simulink model "pulse_heating_single_pack_v03"  (R2025b)
settings: Solver=ode23t  StartTime=0.0  StopTime=1  MaxStep=1e-4  RelTol=1e-3
undefined symbols (not defined in the file or in its folder): DiscIntNeverNeededParam
libraries: fl_lib x6, nesl_utility x5, ee_lib x4, batt_lib x1
settings Model: Creator=ADMIN  LastModifiedBy=ADMIN

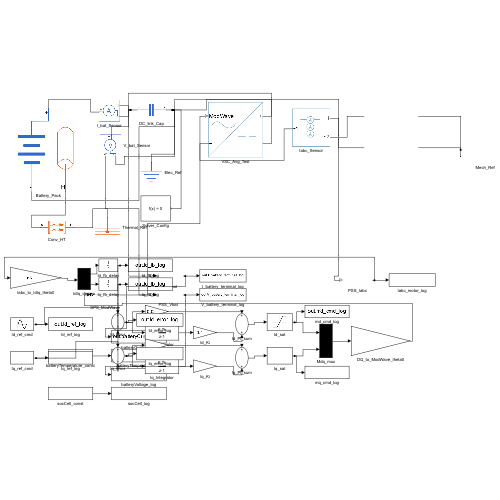
[thumbnail: Simulink's stored preview of the top-level diagram]
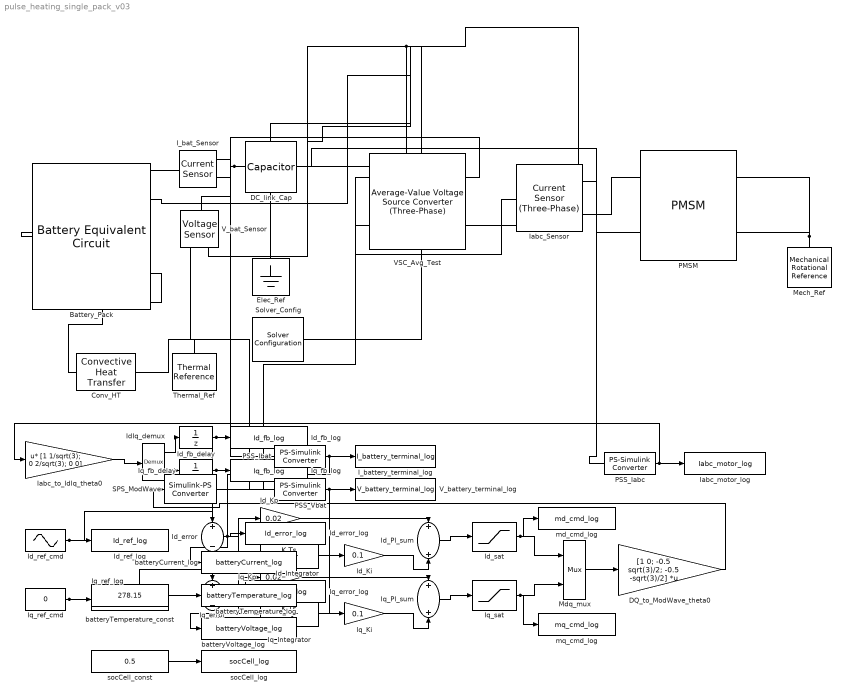
== system pulse_heating_single_pack_v03 ==
  Battery_Pack : batt_lib/Cells/Battery Equivalent Circuit  BatteryCapacity=27 A*hr  ThermalModel=simscape.battery.enum.cells.BatteryThermalModel.LumpedThermalMass  ExtrapolationMethod=simscape.enum.extrapolation.nearest  SOCBreakpoints=[0 0.1 0.25 0.5 0.75 0.9 1]  TemperatureBreakpoints=[278 293 313] K  OpenCircuitVoltage=[757.2312 770.256 784.8792 801.9432 847.9944 880.7832 905.6448] V  OpenCircuitVoltageThermal=[753.84 756 758.16;766.8 771.12 768.96;781.92 784.08 786.24;801.36 801.36 803.52;844.56 848.88 851.04;879.12 881.28 881.28;905.04 905.04 905.04] V  VoltageRange=[0, inf] V  HysteresisModel=simscape.battery.enum.cells.HysteresisModel.none  MaximumHysteresisVoltage=[0, 0, 0, 0, 0, 0, 0] V  InstantaneousHysteresisVoltage=[0, 0, 0, 0, 0, 0, 0] V  HysteresisRate=0.1  MaximumHysteresisVoltageThermal=[0, 0, 0; 0, 0, 0; 0, 0, 0; 0, 0, 0; 0, 0, 0; 0, 0, 0; 0, 0, 0] V  InstantaneousHysteresisVoltageThermal=[0, 0, 0; 0, 0, 0; 0, 0, 0; 0, 0, 0; 0, 0, 0; 0, 0, 0; 0, 0, 0] V  HysteresisRateThermal=0.1  ResistanceSOCBreakpoints=[0, .1, .25, .5, .75, .9, 1]  ResistanceTemperatureBreakpoints=[278, 293, 313] K  ResistanceCurrentBreakpoints=[-1 0 1] A  CurrentDependence=simscape.battery.enum.cells.CurrentDependence.Disabled  R0=[1.836 1.836 1.8792 1.7712 1.7928 1.836 1.836] Ohm  R0I=[2.5272 1.836 1.944;2.376 1.836 1.944;2.4624 1.8792 1.9872;2.3112 1.7712 1.9008;2.3112 1.7928 1.9656;2.4408 1.836 1.9224;2.5056 1.836 1.9224] Ohm  R0Thermal=[2.5272 1.836 1.944;2.376 1.836 1.944;2.4624 1.8792 1.9872;2.3112 1.7712 1.9008;2.3112 1.7928 1.9656;2.4408 1.836 1.9224;2.5056 1.836 1.9224] Ohm  R0ThermalI=repmat([2.5272 1.836 1.944;2.376 1.836 1.944;2.4624 1.8792 1.9872;2.3112 1.7712 1.9008;2.3112 1.7928 1.9656;2.4408 1.836 1.9224;2.5056 1.836 1.9224], 1, 1, 3) Ohm  DischargeR0=[.0085, .0085, .0087, .0082, .0083, .0085, .0085] Ohm  ChargeR0=[.0085, .0085, .0087, .0082, .0083, .0085, .0085] Ohm  ChargeR0Thermal=[.0117, .0085, .009; .011, .0085, .009; .0114, .0087, .0092; .0107, .0082, .0088; .0107, .0083, .0091; .0113, .0085, .0089; .0116, .0085, .0089] Ohm  DischargeR0Thermal=[.0117, .0085, .009; .011, .0085, .009; .0114, .0087, .0092; .0107, .0082, .0088; .0107, .0083, .0091; .0113, .0085, .0089; .0116, .0085, .0089] Ohm  RCPairs=simscape.battery.enum.cells.RCPairs.noDynamics  R1=[.0029, .0024, .0026, .0016, .0023, .0018, .0017] Ohm  Tau1=[36, 45, 105, 29, 77, 33, 39] s  R2=[.0029, .0024, .0026, .0016, .0023, .0018, .0017] Ohm  Tau2=[36, 45, 105, 29, 77, 33, 39] s  R3=[.0029, .0024, .0026, .0016, .0023, .0018, .0017] Ohm  Tau3=[36, 45, 105, 29, 77, 33, 39] s  R1I=[.0109, .0029, .0013; .0069, .0024, .0012; .0047, .0026, .0013; .0034, .0016, .001; .0033, .0023, .0014; .0033, .0018, .0011; .0028, .0017, .0011] Ohm  Tau1I=[20, 36, 39; 31, 45, 39; 109, 105, 61; 36, 29, 26; 59, 77, 67; 40, 33, 29; 25, 39, 33] s  R2I=[.0109, .0029, .0013; .0069, .0024, .0012; .0047, .0026, .0013; .0034, .0016, .001; .0033, .0023, .0014; .0033, .0018, .0011; .0028, .0017, .0011] Ohm  Tau2I=[20, 36, 39; 31, 45, 39; 109, 105, 61; 36, 29, 26; 59, 77, 67; 40, 33, 29; 25, 39, 33] s  R3I=[.0109, .0029, .0013; .0069, .0024, .0012; .0047, .0026, .0013; .0034, .0016, .001; .0033, .0023, .0014; .0033, .0018, .0011; .0028, .0017, .0011] Ohm  Tau3I=[20, 36, 39; 31, 45, 39; 109, 105, 61; 36, 29, 26; 59, 77, 67; 40, 33, 29; 25, 39, 33] s  DischargeR1=[0.6264 0.5184 0.5616 0.3456 0.4968 0.3888 0.3672] Ohm  DischargeTau1=[36 45 105 29 77 33 39] s  ChargeR1=[0.6264 0.5184 0.5616 0.3456 0.4968 0.3888 0.3672] Ohm  ChargeTau1=[36 45 105 29 77 33 39] s  DischargeR2=[0.6264 0.5184 0.5616 0.3456 0.4968 0.3888 0.3672] Ohm  DischargeTau2=[36 45 105 29 77 33 39] s  ChargeR2=[0.6264 0.5184 0.5616 0.3456 0.4968 0.3888 0.3672] Ohm  ChargeTau2=[36 45 105 29 77 33 39] s  DischargeR3=[0.6264 0.5184 0.5616 0.3456 0.4968 0.3888 0.3672] Ohm  DischargeTau3=[36 45 105 29 77 33 39] s  ChargeR3=[0.6264 0.5184 0.5616 0.3456 0.4968 0.3888 0.3672] Ohm  ChargeTau3=[36 45 105 29 77 33 39] s  R1Thermal=[.0109, .0029, .0013; .0069, .0024, .0012; .0047, .0026, .0013; .0034, .0016, .001; .0033, .0023, .0014; .0033, .0018, .0011; .0028, .0017, .0011] Ohm  Tau1Thermal=[20, 36, 39; 31, 45, 39; 109, 105, 61; 36, 29, 26; 59, 77, 67; 40, 33, 29; 25, 39, 33] s  R2Thermal=[.0109, .0029, .0013; .0069, .0024, .0012; .0047, .0026, .0013; .0034, .0016, .001; .0033, .0023, .0014; .0033, .0018, .0011; .0028, .0017, .0011] Ohm  Tau2Thermal=[20, 36, 39; 31, 45, 39; 109, 105, 61; 36, 29, 26; 59, 77, 67; 40, 33, 29; 25, 39, 33] s  R3Thermal=[.0109, .0029, .0013; .0069, .0024, .0012; .0047, .0026, .0013; .0034, .0016, .001; .0033, .0023, .0014; .0033, .0018, .0011; .0028, .0017, .0011] Ohm  Tau3Thermal=[20, 36, 39; 31, 45, 39; 109, 105, 61; 36, 29, 26; 59, 77, 67; 40, 33, 29; 25, 39, 33] s  R1ThermalI=repmat([.0109, .0029, .0013; .0069, .0024, .0012; .0047, .0026, .0013; .0034, .0016, .001; .0033, .0023, .0014; .0033, .0018, .0011; .0028, .0017, .0011], 1, 1, 3) Ohm  Tau1ThermalI=repmat([20, 36, 39; 31, 45, 39; 109, 105, 61; 36, 29, 26; 59, 77, 67; 40, 33, 29; 25, 39, 33], 1, 1, 3) s  R2ThermalI=repmat([.0109, .0029, .0013; .0069, .0024, .0012; .0047, .0026, .0013; .0034, .0016, .001; .0033, .0023, .0014; .0033, .0018, .0011; .0028, .0017, .0011], 1, 1, 3) Ohm  Tau2ThermalI=repmat([20, 36, 39; 31, 45, 39; 109, 105, 61; 36, 29, 26; 59, 77, 67; 40, 33, 29; 25, 39, 33], 1, 1, 3) s  R3ThermalI=repmat([.0109, .0029, .0013; .0069, .0024, .0012; .0047, .0026, .0013; .0034, .0016, .001; .0033, .0023, .0014; .0033, .0018, .0011; .0028, .0017, .0011], 1, 1, 3) Ohm  Tau3ThermalI=repmat([20, 36, 39; 31, 45, 39; 109, 105, 61; 36, 29, 26; 59, 77, 67; 40, 33, 29; 25, 39, 33], 1, 1, 3) s  DischargeR1Thermal=[2.3544 0.6264 0.2808;1.4904 0.5184 0.2592;1.0152 0.5616 0.2808;0.7344 0.3456 0.216;0.7128 0.4968 0.3024;0.7128 0.3888 0.2376;0.6048 0.3672 0.2376] Ohm  DischargeTau1Thermal=[20 36 39;31 45 39;109 105 61;36 29 26;59 77 67;40 33 29;25 39 33] s  ChargeR1Thermal=[2.3544 0.6264 0.2808;1.4904 0.5184 0.2592;1.0152 0.5616 0.2808;0.7344 0.3456 0.216;0.7128 0.4968 0.3024;0.7128 0.3888 0.2376;0.6048 0.3672 0.2376] Ohm  ChargeTau1Thermal=[20 36 39;31 45 39;109 105 61;36 29 26;59 77 67;40 33 29;25 39 33] s  DischargeR2Thermal=[2.3544 0.6264 0.2808;1.4904 0.5184 0.2592;1.0152 0.5616 0.2808;0.7344 0.3456 0.216;0.7128 0.4968 0.3024;0.7128 0.3888 0.2376;0.6048 0.3672 0.2376] Ohm  DischargeTau2Thermal=[20 36 39;31 45 39;109 105 61;36 29 26;59 77 67;40 33 29;25 39 33] s  ChargeR2Thermal=[2.3544 0.6264 0.2808;1.4904 0.5184 0.2592;1.0152 0.5616 0.2808;0.7344 0.3456 0.216;0.7128 0.4968 0.3024;0.7128 0.3888 0.2376;0.6048 0.3672 0.2376] Ohm  ChargeTau2Thermal=[20 36 39;31 45 39;109 105 61;36 29 26;59 77 67;40 33 29;25 39 33] s  DischargeR3Thermal=[2.3544 0.6264 0.2808;1.4904 0.5184 0.2592;1.0152 0.5616 0.2808;0.7344 0.3456 0.216;0.7128 0.4968 0.3024;0.7128 0.3888 0.2376;0.6048 0.3672 0.2376] Ohm  DischargeTau3Thermal=[20 36 39;31 45 39;109 105 61;36 29 26;59 77 67;40 33 29;25 39 33] s  ChargeR3Thermal=[2.3544 0.6264 0.2808;1.4904 0.5184 0.2592;1.0152 0.5616 0.2808;0.7344 0.3456 0.216;0.7128 0.4968 0.3024;0.7128 0.3888 0.2376;0.6048 0.3672 0.2376] Ohm  ChargeTau3Thermal=[20 36 39;31 45 39;109 105 61;36 29 26;59 77 67;40 33 29;25 39 33] s  SelfDischargeResistor=simscape.battery.enum.cells.BatteryEnable.Disabled  SelfDischargeR=7e3 Ohm  SelfDischargeRThermal=[8000, 7000, 6000] Ohm  CyclingAgingMethod=simscape.battery.enum.cells.CyclingAgingMethod.disabled  CycleCalculationMethod=simscape.battery.enum.cells.CycleCalculationMethod.EquivalentCycles  NumDisCycles=100  OCVChange=0  R0Change=0  CapacityChange=0  SelfDischargeRChange=0  R1Change=0  R2Change=0  R3Change=0  NumDisCyclesBreakpoints=[0, 100, 200, 300]  AgingTemperatureBreakpoints=[298.15, 323.15] K  AgingCurrentBreakpoints=[-.1, -.5, -5] A  OCVChangeVec=[0, 0, 0, 0]  OCVChangeThermal=[0, 0; 0, 0; 0, 0; 0, 0]  R0ChangeVec=[0, 0, 0, 0]  R0ChangeThermal=[0, 0; 0, 0; 0, 0; 0, 0]  R0ChangeThermalI=repmat(0, 4, 2, 3)  R0CyclingChangeInitialTarget=0  CapacityChangeVec=[0, 0, 0, 0]  CapacityChangeThermal=[0, 0; 0, 0; 0, 0; 0, 0]  CapacityChangeThermalI=repmat(0, 4, 2, 3)  CapacityCyclingChangeInitialTarget=0  SelfDischargeRChangeVec=[0, 0, 0, 0]  SelfDischargeRChangeThermal=[0, 0; 0, 0; 0, 0; 0, 0]  SelfDischargeRChangeThermalI=repmat(0, 4, 2, 3)  SelfDischargeRCyclingChangeInitialTarget=0  R1ChangeVec=[0, 0, 0, 0]  R1ChangeThermal=[0, 0; 0, 0; 0, 0; 0, 0]  R1ChangeThermalI=repmat(0, 4, 2, 3)  R1CyclingChangeInitialTarget=0  R2ChangeVec=[0, 0, 0, 0]  R2ChangeThermal=[0, 0; 0, 0; 0, 0; 0, 0]  R2ChangeThermalI=repmat(0, 4, 2, 3)  R2CyclingChangeInitialTarget=0  R3ChangeVec=[0, 0, 0, 0]  R3ChangeThermal=[0, 0; 0, 0; 0, 0; 0, 0]  R3ChangeThermalI=repmat(0, 4, 2, 3)  R3CyclingChangeInitialTarget=0  CalendarAgeResistance=simscape.battery.enum.cells.BatteryEnable.Disabled  CalendarAgeCapacity=simscape.battery.enum.cells.BatteryEnable.Disabled  CalendarAgingMethod=simscape.battery.enum.cells.CalendarAgingMethod.equation  StorageVariable=simscape.battery.enum.cells.StorageVariable.OCV  OCVDuringStorage=0.9  SOCDuringStorage=0.6  StorageTimeIntervals=[0] d  StorageTemperatures=[273] K  ResistanceScalingOCV=2.2134e6  ResistanceScalingOCVOffset=1.632e6  ResistanceExponentialIncrease=0.515833569 V  ResistanceTimeExponent=0.75  ResistanceAgeTemperatureBreakpoints=[273.15, 298.15, 323.15] K  ResistanceAgeTimeBreakpoints=[0, 90, 180, 270] d  PercentResistanceChange=[0, 0, 0]  ResistanceTimeBreakpoints=100 d  PercentResistanceChangeThermal=[0, 0, 0; 0, 0, 0; 0, 0, 0; 0, 0, 0]  CapacityScalingOCV=1.5097e07  CapacityScalingOCVOffset=8.3625e06  CapacityExponentialIncrease=0.6011 V  CapacityTimeExponent=0.75  CapacityAgeTemperatureBreakpoints=[273.15, 298.15, 323.15] K  CapacityAgeTimeBreakpoints=[0, 90, 180, 270] d  PercentCapacityChange=[0, 0, 0]  CapacityTimeBreakpoints=100 d  PercentCapacityChangeThermal=[0, 0, 0; 0, 0, 0; 0, 0, 0; 0, 0, 0]  SimulationTemperature=278.15 K  BatteryThermalMass=21600 J/K  NumThermalModels=6  ThermalConductivityZ=18 W/(K*m)  CrossSectionalAreaXY=3.5e-4 m^2  Height=0.07 m  ReversibleHeatModel=simscape.battery.enum.cells.ReversibleHeatModel.Disabled  EntropicCoefficient=[0, 0, 0, 0, 0, 0, 0] mV/K  CurrentDirectionality=simscape.battery.enum.cells.BatteryEnable.Disabled  stateOfCharge_specify=on  stateOfCharge_priority=High  stateOfCharge=0.5  stateOfCharge_nominal_specify=off  stateOfCharge_nominal_value=1  stateOfCharge_nominal_unit=1  batteryVoltage_specify=off  batteryVoltage_priority=None  batteryVoltage=0 V  batteryVoltage_nominal_specify=off  batteryVoltage_nominal_value=1  batteryVoltage_nominal_unit=V  batteryCurrent_specify=off  batteryCurrent_priority=None  batteryCurrent=0 A  batteryCurrent_nominal_specify=off  batteryCurrent_nominal_value=1  batteryCurrent_nominal_unit=A  numCycles_specify=off  numCycles_priority=High  numCycles=0  numCycles_nominal_specify=off  numCycles_nominal_value=1  numCycles_nominal_unit=1  batteryTemperature_specify=on  batteryTemperature_priority=High  batteryTemperature=278.15 K  batteryTemperature_nominal_specify=off  batteryTemperature_nominal_value=1  batteryTemperature_nominal_unit=K  hysteresisState_specify=off  hysteresisState_priority=High  hysteresisState=0  hysteresisState_nominal_specify=off  hysteresisState_nominal_value=1  hysteresisState_nominal_unit=1  isExothermFaulted_specify=off  isExothermFaulted_priority=None  isExothermFaulted=0  isExothermFaulted_nominal_specify=off  isExothermFaulted_nominal_value=1  isExothermFaulted_nominal_unit=1  reactionHeatRate_specify=off  reactionHeatRate_priority=None  reactionHeatRate=0 W  reactionHeatRate_nominal_specify=off  reactionHeatRate_nominal_value=1  reactionHeatRate_nominal_unit=W  reactionExtent_specify=off  reactionExtent_priority=None  reactionExtent=0  reactionExtent_nominal_specify=off  reactionExtent_nominal_value=1  reactionExtent_nominal_unit=1
      settings: InternalSimscapePortConfiguration="{\"Bottom\":[{\"id\":\"n\",\"label\":\"-\",\"type\":\"foundation.electrical.electrical\"},{\"id\":\"H\",\"label\":\"H\",\"type\":\"foundation.thermal.thermal\"}],\"Left\":[],\"Right\":[],\"Top\":[{\"id\":\"p\",\"label\":\"+\",\"type\":\"foundation.electrical.electrical\"}]}"
  Conv_HT : fl_lib/Thermal/Thermal Elements/Convective Heat Transfer  thermal_type=foundation.enum.constant_variable.constant  area=1e-4 m^2  heat_tr_coeff=20 W/(K*m^2)  min_heat_tr_coeff=1e-3 W/(K*m^2)  T_specify=off  T_priority=None  T=0 K  T_nominal_specify=off  T_nominal_value=1  T_nominal_unit=K  Q_specify=off  Q_priority=None  Q=0 W  Q_nominal_specify=off  Q_nominal_value=1  Q_nominal_unit=W
  DC_link_Cap : ee_lib/Passive/Capacitor  cap_option=ee.enum.passive.capacitor.capOption.const  c=1e-3 F  Cvec=[1e-05, 1e-06] F  Vvec=[0, 10] V  CV_table_symmetry=ee.enum.passive.capacitor.tableSymmetry.yes  f_vec=[1, 10] kHz  DFext_vec=[.8, 1.2]  enable_C_tol=ee.enum.toleranceApplication.none  averaging_period=0 s  C_tol=5  tol_distribution=ee.enum.toleranceDistribution.uniform  nSigma=4  r=0 Ohm  g=0 1/Ohm  enable_operating_limits=ee.enum.enable.no  operating_limit_action=ee.enum.passive.reportOpLim.warn  max_working_voltage_range=[-25, 25] V  power_rating=1 W  maxTemperature=85 degC  thermalEnable=false  thermalMass=1 J/K  i_specify=off  i_priority=None  i=0 A  i_nominal_specify=off  i_nominal_value=1  i_nominal_unit=A  v_specify=off  v_priority=None  v=0 V  v_nominal_specify=off  v_nominal_value=1  v_nominal_unit=V  vc_specify=on  vc_priority=High  vc=801.9432 V  vc_nominal_specify=off  vc_nominal_value=1  vc_nominal_unit=V  T_specify=off  T_priority=None  T=298.15 K  T_nominal_specify=off  T_nominal_value=1  T_nominal_unit=K
  DQ_to_ModWave_theta0 : Gain  Gain=[1 0; -0.5 sqrt(3)/2; -0.5 -sqrt(3)/2]  Multiplication=Matrix(K*u)
  Elec_Ref : fl_lib/Electrical/Electrical Elements/Electrical Reference
  I_bat_Sensor : fl_lib/Electrical/Electrical Sensors/Current Sensor
  I_battery_terminal_log : ToWorkspace  VariableName=I_battery_terminal_log  SaveFormat=Timeseries  SampleTime=-1
  Iabc_Sensor : ee_lib/Sensors & Transducers/Current Sensor (Three-Phase)
  Iabc_motor_log : ToWorkspace  VariableName=Iabc_motor_log  SaveFormat=Timeseries  SampleTime=-1
  Iabc_to_IdIq_theta0 : Gain  Gain=[1 1/sqrt(3); 0 2/sqrt(3); 0 0]  Multiplication=Matrix(u*K)
  IdIq_demux : Demux  Outputs=2
  Id_Integrator : DiscreteIntegrator  SampleTime=1e-4  ICPrevOutput=DiscIntNeverNeededParam  ICPrevScaledInput=DiscIntNeverNeededParam
  Id_Ki : Gain  Gain=0.1
  Id_Kp : Gain  Gain=0.02
  Id_PI_sum : Sum
  Id_error : Sum  Inputs=+-
  Id_error_log : ToWorkspace  VariableName=Id_error_log  SaveFormat=Timeseries  SampleTime=-1
  Id_fb_delay : UnitDelay  SampleTime=1e-4  HasFrameUpgradeWarning=on
  Id_fb_log : ToWorkspace  VariableName=Id_fb_log  SaveFormat=Timeseries  SampleTime=-1
  Id_ref_cmd : Sin  Amplitude=20  Frequency=2*pi*1250  SampleTime=0
  Id_ref_log : ToWorkspace  VariableName=Id_ref_log  SaveFormat=Timeseries  SampleTime=-1
  Id_sat : Saturate  UpperLimit=0.2  LowerLimit=-0.2
  Iq_Integrator : DiscreteIntegrator  SampleTime=1e-4  ICPrevOutput=DiscIntNeverNeededParam  ICPrevScaledInput=DiscIntNeverNeededParam
  Iq_Ki : Gain  Gain=0.1
  Iq_Kp : Gain  Gain=0.02
  Iq_PI_sum : Sum
  Iq_error : Sum  Inputs=+-
  Iq_error_log : ToWorkspace  VariableName=Iq_error_log  SaveFormat=Timeseries  SampleTime=-1
  Iq_fb_delay : UnitDelay  SampleTime=1e-4  HasFrameUpgradeWarning=on
  Iq_fb_log : ToWorkspace  VariableName=Iq_fb_log  SaveFormat=Timeseries  SampleTime=-1
  Iq_ref_cmd : Constant  Value=0
  Iq_ref_log : ToWorkspace  VariableName=Iq_ref_log  SaveFormat=Timeseries  SampleTime=-1
  Iq_sat : Saturate  UpperLimit=0.2  LowerLimit=-0.2
  Mdq_mux : Mux  Inputs=2
  Mech_Ref : fl_lib/Mechanical/Rotational Elements/Mechanical Rotational Reference
  PMSM : ee_lib/Electromechanical/Permanent Magnet/PMSM  port_option=ee.enum.threePhasePort.composite  winding_type=ee.enum.electromech.statorconfiguration.wye  machine_param=ee.enum.pmsm.parameterization.constant  nPolePairs=6  pmflux_param=ee.enum.pmflux.fluxlinkage  pm_flux_linkage=0.03 Wb  torque_constant=0.18 N*m/A  back_emf_constant=0.18 V*s/rad  stator_param=ee.enum.statorparam.LdLqL0  Ld=0.00019 H  Lq=0.00025 H  idVec=[-200, 0, 200] A  iqVec=[-200, 0, 200] A  LdMatrix=0.0002 * ones(3, 3) H  LqMatrix=0.0002 * ones(3, 3) H  PmMatrix=0.1 * ones(3, 3) Wb  ktMatrix=0.18 * ones(3, 3) N*m/A  keMatrix=0.18 * ones(3, 3) V*s/rad  L0=0.00016 H  Ls=0.0002 H  Lm=-0.00002 H  Ms=0.00002 H  Rs=0.013 Ohm  zero_sequence=ee.enum.park.zerosequence.include  axes_param=ee.enum.rotorangle.daxis  loss_param=ee.enum.ironloss.none  losses_oc=[0, 0, 0] W  losses_sc=[0, 0, 0] W  f_losses=60 Hz  Isc_losses=95 A  J=0.01 kg*m^2  lam=0 N*m*s/rad  i_d_specify=off  i_d_priority=None  i_d=0 A  i_d_nominal_specify=off  i_d_nominal_value=1  i_d_nominal_unit=A  i_q_specify=off  i_q_priority=None  i_q=0 A  i_q_nominal_specify=off  i_q_nominal_value=1  i_q_nominal_unit=A  torque_specify=off  torque_priority=None  torque=0 N*m  torque_nominal_specify=off  torque_nominal_value=1  torque_nominal_unit=N*m  angular_velocity_specify=off  angular_velocity_priority=High  angular_velocity=0 rpm  angular_velocity_nominal_specify=off  angular_velocity_nominal_value=1  angular_velocity_nominal_unit=rpm  angular_position_specify=off  angular_position_priority=High  angular_position=0 deg  angular_position_nominal_specify=off  angular_position_nominal_value=1  angular_position_nominal_unit=deg  alpha=3.93e-3 1/K  alpha_flux=-0.001 1/K  Tmeas=298.15 K  stator_thermal_mass=100 J/K  rotor_thermal_mass=200 J/K  Rm_percent_rotor=90  Rd_percent_rotor=30  temperatureA_specify=off  temperatureA_priority=High  temperatureA=25 degC  temperatureA_nominal_specify=off  temperatureA_nominal_value=1  temperatureA_nominal_unit=degC  temperatureB_specify=off  temperatureB_priority=High  temperatureB=25 degC  temperatureB_nominal_specify=off  temperatureB_nominal_value=1  temperatureB_nominal_unit=degC  temperatureC_specify=off  temperatureC_priority=High  temperatureC=25 degC  temperatureC_nominal_specify=off  temperatureC_nominal_value=1  temperatureC_nominal_unit=degC  temperatureR_specify=off  temperatureR_priority=High  temperatureR=25 degC  temperatureR_nominal_specify=off  temperatureR_nominal_value=1  temperatureR_nominal_unit=degC
      settings: InternalSimscapePortConfiguration="{\"Bottom\":[],\"Left\":[{\"id\":\"N\",\"label\":\"~\",\"type\":\"foundation.electrical.three_phase\"},{\"id\":\"n\",\"label\":\"n\",\"type\":\"foundation.electrical.electrical\"}],\"Right\":[{\"id\":\"R\",\"label\":\"R\",\"type\":\"foundation.mechanical.rotational.rotational\"},{\"id\":\"C\",\"label\":\"C\",\"type\":\"foundation.mechanical.rotational.rotational\"}],\"Top\":[]}"
  PSS_Iabc : nesl_utility/PS-Simulink Converter  PhysicalDomain=network_engine_domain  SubClassName=ps_output  LeftPortType=input  RightPortType=output  PseudoPeriodic=off  Frequencies=[]  VectorFormat=inherit  Unit=inherit  AffineConversion=off
  PSS_Ibat : nesl_utility/PS-Simulink Converter  PhysicalDomain=network_engine_domain  SubClassName=ps_output  LeftPortType=input  RightPortType=output  PseudoPeriodic=off  Frequencies=[]  VectorFormat=inherit  Unit=inherit  AffineConversion=off
  PSS_Vbat : nesl_utility/PS-Simulink Converter  PhysicalDomain=network_engine_domain  SubClassName=ps_output  LeftPortType=input  RightPortType=output  PseudoPeriodic=off  Frequencies=[]  VectorFormat=inherit  Unit=inherit  AffineConversion=off
  SPS_ModWave : nesl_utility/Simulink-PS Converter  PhysicalDomain=network_engine_domain  SubClassName=ps_input  LeftPortType=input  RightPortType=output  PseudoPeriodic=off  Frequencies=[]  NoiseDistribution=none  NoiseParameters=[]  Unit=1  AffineConversion=off  FilteringAndDerivatives=provide  SimscapeFilterOrder=1  InputFilterTimeConstant=0.001  UdotUserProvided=0
  Solver_Config : nesl_utility/Solver Configuration  PhysicalDomain=network_engine_domain  SubClassName=solver  LeftPortType=input  RightPortType=generic  Tones=[]  Harmonics=[]  SimulateNoise=off  Profile=off  UseLocalSampling=off  EnableSwitchedLinearOptims=on  FrequencyDomain=off  UseCCode=off  RelTol=0.001  AbsTol=0.001  MinStep=1e-09  ToWorkspace=off  RevertToSquareIcSolve=off  NumHomotopyIterations=100  PhasorMode=off  PhasorModeNumHarmonics=1  ConsistencySolver=NEWTON_XTOL_AFTER_FTOL  IndexReductionMethod=DerivativeReplacement  DoDC=off  ResidualTolerance=1e-09  ConsistencyTolSource=GLOBAL  ConsistencyAbsTol=0.001  ConsistencyRelTol=0.001  ConsistencyTolFactor=0.001  UseLocalSolver=off  LocalSolverChoice=NE_BACKWARD_EULER_ADVANCER  ResolveIndetEquations=on  FunctionEvalNumThread=1  LocalSolverSampleTime=0.001  DoFixedCost=off  MaxNonlinIter=3  MaxModeIter=2  ComputeImpulses=off  ImpulseIterations=2  LinearAlgebra=auto  LinearAlgebraNumThread=0  EquationFormulation=NE_TIME_EF  DelaysMemoryBudget=1024  AutomaticFiltering=on  FilteringTimeConstant=0.001  PartitionStorageMethod=AS_NEEDED  PartitionMemoryBudget=1024  PartitionMethod=ROBUST  MultibodyUseLocalSolver=off  MultibodyLocalSolverChoice=ODE1  MultibodyLocalSolverSampleTime=0.001
  Thermal_Ref : fl_lib/Thermal/Thermal Elements/Thermal Reference
  VSC_Avg_Test : ee_lib/Semiconductors & Converters/Converters/Average-Value Voltage Source Converter (Three-Phase)  port_option=ee.enum.threePhasePort.composite  frequency_option=ee.enum.converters.frequency.variable  input_option=Modulation waveforms  FRated=60 Hz  losses_parameterization=ee.enum.converters.losses.fixed  Pfixed=1 W  ks=0.01  kc1=1.7 V  kc2=0.01 Ohm  Ploss_vect=[100, 800, 1870, 3250, 4900] W  Irms_vect=[10, 100, 200, 300, 400] A  Vdc_nom=300 V  thermal_mass=30000 J/K  temperature_specify=off  temperature_priority=High  temperature=298.15 K  temperature_nominal_specify=off  temperature_nominal_value=1  temperature_nominal_unit=K
      settings: InternalSimscapePortConfiguration="{\"Bottom\":[],\"Left\":[{\"id\":\"ModWave\",\"label\":\"ModWave\",\"type\":\"input\"},{\"id\":\"N\",\"label\":\"~\",\"type\":\"foundation.electrical.three_phase\"}],\"Right\":[{\"id\":\"p\",\"label\":\"+\",\"type\":\"foundation.electrical.electrical\"},{\"id\":\"n\",\"label\":\"-\",\"type\":\"foundation.electrical.electrical\"}],\"Top\":[]}"
  V_bat_Sensor : fl_lib/Electrical/Electrical Sensors/Voltage Sensor
  V_battery_terminal_log : ToWorkspace  VariableName=V_battery_terminal_log  SaveFormat=Timeseries  SampleTime=-1
  batteryCurrent_log : ToWorkspace  VariableName=batteryCurrent_log  SaveFormat=Timeseries  SampleTime=-1
  batteryTemperature_const : Constant  Value=278.15
  batteryTemperature_log : ToWorkspace  VariableName=batteryTemperature_log  SaveFormat=Timeseries  SampleTime=-1
  batteryVoltage_log : ToWorkspace  VariableName=batteryVoltage_log  SaveFormat=Timeseries  SampleTime=-1
  md_cmd_log : ToWorkspace  VariableName=md_cmd_log  SaveFormat=Timeseries  SampleTime=-1
  mq_cmd_log : ToWorkspace  VariableName=mq_cmd_log  SaveFormat=Timeseries  SampleTime=-1
  socCell_const : Constant  Value=0.5
  socCell_log : ToWorkspace  VariableName=socCell_log  SaveFormat=Timeseries  SampleTime=-1
  wires:
  PSS_Ibat/1 -> I_battery_terminal_log/1, batteryCurrent_log/1
  PSS_Vbat/1 -> V_battery_terminal_log/1, batteryVoltage_log/1
  PSS_Iabc/1 -> Iabc_motor_log/1, Iabc_to_IdIq_theta0/1
  batteryTemperature_const/1 -> batteryTemperature_log/1
  socCell_const/1 -> socCell_log/1
  Iabc_to_IdIq_theta0/1 -> IdIq_demux/1
  IdIq_demux/1 -> Id_fb_delay/1
  IdIq_demux/2 -> Iq_fb_delay/1
  Id_fb_delay/1 -> Id_error/2, Id_fb_log/1
  Iq_fb_delay/1 -> Iq_error/2, Iq_fb_log/1
  Id_ref_cmd/1 -> Id_error/1, Id_ref_log/1
  Iq_ref_cmd/1 -> Iq_error/1, Iq_ref_log/1
  Id_error/1 -> Id_Kp/1, Id_Integrator/1, Id_error_log/1
  Id_Kp/1 -> Id_PI_sum/1
  Id_Integrator/1 -> Id_Ki/1
  Id_Ki/1 -> Id_PI_sum/2
  Id_PI_sum/1 -> Id_sat/1
  Id_sat/1 -> Mdq_mux/1, md_cmd_log/1
  Iq_error/1 -> Iq_Kp/1, Iq_Integrator/1, Iq_error_log/1
  Iq_Kp/1 -> Iq_PI_sum/1
  Iq_Integrator/1 -> Iq_Ki/1
  Iq_Ki/1 -> Iq_PI_sum/2
  Iq_PI_sum/1 -> Iq_sat/1
  Iq_sat/1 -> Mdq_mux/2, mq_cmd_log/1
  Mdq_mux/1 -> DQ_to_ModWave_theta0/1
  DQ_to_ModWave_theta0/1 -> SPS_ModWave/1
  connections:
  Battery_Pack/LConn1 -- I_bat_Sensor/LConn1
  I_bat_Sensor/RConn2 -- VSC_Avg_Test/RConn1 -- DC_link_Cap/LConn1 -- V_bat_Sensor/LConn1
  Battery_Pack/RConn1 -- VSC_Avg_Test/RConn2 -- V_bat_Sensor/RConn2 -- Elec_Ref/LConn1 -- Solver_Config/RConn1 -- DC_link_Cap/RConn1 -- PMSM/LConn2
  Battery_Pack/RConn2 -- Conv_HT/LConn1
  Conv_HT/RConn1 -- Thermal_Ref/LConn1
  SPS_ModWave/RConn1 -- VSC_Avg_Test/LConn1
  VSC_Avg_Test/LConn2 -- Iabc_Sensor/LConn1
  Iabc_Sensor/RConn2 -- PMSM/LConn1
  Mech_Ref/LConn1 -- PMSM/RConn1 -- PMSM/RConn2
  I_bat_Sensor/RConn1 -- PSS_Ibat/LConn1
  V_bat_Sensor/RConn1 -- PSS_Vbat/LConn1
  Iabc_Sensor/RConn1 -- PSS_Iabc/LConn1
